simulink model "EKF_sim"  (R2020a)
settings: Solver=VariableStepAuto  StartTime=0.0  StopTime=257  RelTol=1e-3
values from neighbouring files (symbols this model uses):
  acc_variance = 4.8e-2    (= 0.048)    [init.m]
  bias_acc_variance = 4e-14    [init.m]
  bias_gyro_variance = 4e-14    [init.m]
  Delta2 = [260.168 -23.8158 1.64305]    [init.m]
  DT = EKF_DT    (= 0.01)    [init.m]
  EKF_DT = 0.01    [init.m]
  g = 9.81    [init.m]
  GPS_variance = 5    [init.m]
  gyro_variance = 4.8e-6    (= 4.8e-06)    [init.m]
  h0 = 38.8887000000000000    (= 38.8887)    [init.m]
  head_variance = 5e-2    (= 0.05)    [init.m]
  init_time = 4    [init.m]
  lambda_xa = 1e-4    (= 0.0001)    [init.m]
  lambda_xg = 1e-3    (= 0.001)    [init.m]
  lat0 = 36.7144590750000006    (= 36.714459075)    [init.m]
  lon0 = -4.4789588283333330    (= -4.47895882833)    [init.m]
  SHOE_buffer_N = 100    [init.m]
  SHOE_threshold = 2000    [init.m]
  t1_end = 100    [init.m]
  t1_start = 90    [init.m]
  t2_end = 193    [init.m]
  t2_start = 183    [init.m]
  t3_end = 213    [init.m]
  t3_start = 203    [init.m]
  t4_end = 244    [init.m]
  t4_start = 237    [init.m]
  type_of_GPS = 1    [init.m]
  vel_variance = 1e-2    (= 0.01)    [init.m]
  zero_vel_period = 0.1    [init.m]
(part 1 of 5)
settings Model: PauseTimes=232.9  Creator=Marco  LastModifiedBy=Marco

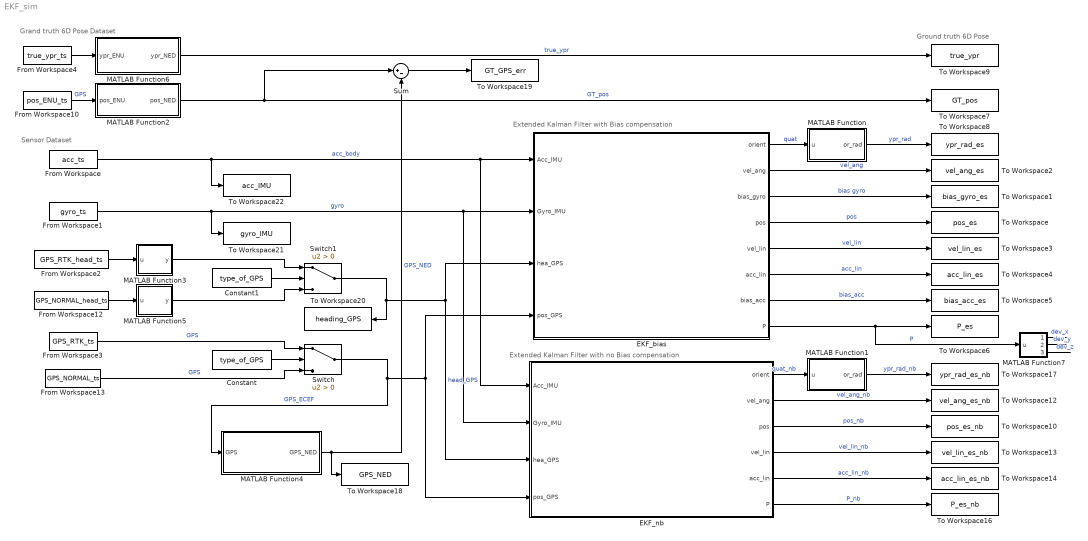
== system EKF_sim ==
  note: Grand truth 6D Pose Dataset
  note: Ground truth 6D Pose
  note: Sensor Dataset
  note: Extended Kalman Filter with Bias compensation
  note: Extended Kalman Filter with no Bias compensation
  Constant : Constant  Value=type_of_GPS
  Constant1 : Constant  Value=type_of_GPS
  EKF_bias : Subsystem
  EKF_nb : Subsystem
  From Workspace : FromWorkspace  VariableName=acc_ts  SampleTime=EKF_DT  OutputAfterFinalValue=Holding final value
  From Workspace1 : FromWorkspace  VariableName=gyro_ts  SampleTime=EKF_DT  OutputAfterFinalValue=Holding final value
  From Workspace10 : FromWorkspace  VariableName=pos_ENU_ts  SampleTime=0.01  OutputAfterFinalValue=Holding final value
  From Workspace12 : FromWorkspace  VariableName=GPS_NORMAL_head_ts  SampleTime=1  Interpolate=off  OutputAfterFinalValue=Holding final value
  From Workspace13 : FromWorkspace  VariableName=GPS_NORMAL_ts  SampleTime=1  Interpolate=off  OutputAfterFinalValue=Holding final value
  From Workspace2 : FromWorkspace  VariableName=GPS_RTK_head_ts  SampleTime=0.25  OutputAfterFinalValue=Holding final value
  From Workspace3 : FromWorkspace  VariableName=GPS_RTK_ts  SampleTime=0.25  OutputAfterFinalValue=Holding final value
  From Workspace4 : FromWorkspace  VariableName=true_ypr_ts  SampleTime=EKF_DT  OutputAfterFinalValue=Holding final value
  MATLAB Function : MATLAB Function  TreatAsAtomicUnit=on
  MATLAB Function1 : MATLAB Function  TreatAsAtomicUnit=on
  MATLAB Function2 : MATLAB Function  TreatAsAtomicUnit=on
  MATLAB Function3 : MATLAB Function  TreatAsAtomicUnit=on
  MATLAB Function4 : MATLAB Function  TreatAsAtomicUnit=on
  MATLAB Function5 : MATLAB Function  TreatAsAtomicUnit=on
  MATLAB Function6 : MATLAB Function  TreatAsAtomicUnit=on
  MATLAB Function7 : MATLAB Function  TreatAsAtomicUnit=on
  Sum : Sum  Inputs=|+-
  Switch : Switch  Criteria=u2 > Threshold
  Switch1 : Switch  Criteria=u2 > Threshold
  To Workspace : ToWorkspace  VariableName=pos_es  SaveFormat=Timeseries  SampleTime=-1
  To Workspace1 : ToWorkspace  VariableName=bias_gyro_es  SaveFormat=Timeseries  SampleTime=-1
  To Workspace10 : ToWorkspace  VariableName=pos_es_nb  SaveFormat=Timeseries  SampleTime=-1
  To Workspace12 : ToWorkspace  VariableName=vel_ang_es_nb  SaveFormat=Timeseries  SampleTime=-1
  To Workspace13 : ToWorkspace  VariableName=vel_lin_es_nb  SaveFormat=Timeseries  SampleTime=-1
  To Workspace14 : ToWorkspace  VariableName=acc_lin_es_nb  SaveFormat=Timeseries  SampleTime=-1
  To Workspace16 : ToWorkspace  VariableName=P_es_nb  SaveFormat=Timeseries  SampleTime=-1
  To Workspace17 : ToWorkspace  VariableName=ypr_rad_es_nb  SaveFormat=Timeseries  SampleTime=-1
  To Workspace18 : ToWorkspace  VariableName=GPS_NED  SaveFormat=Timeseries  SampleTime=-1
  To Workspace19 : ToWorkspace  VariableName=GT_GPS_err  SaveFormat=Timeseries  SampleTime=-1
  To Workspace2 : ToWorkspace  VariableName=vel_ang_es  SaveFormat=Timeseries  SampleTime=-1
  To Workspace20 : ToWorkspace  VariableName=heading_GPS  SaveFormat=Timeseries  SampleTime=-1
  To Workspace21 : ToWorkspace  VariableName=gyro_IMU  SaveFormat=Timeseries  SampleTime=-1
  To Workspace22 : ToWorkspace  VariableName=acc_IMU  SaveFormat=Timeseries  SampleTime=-1
  To Workspace3 : ToWorkspace  VariableName=vel_lin_es  SaveFormat=Timeseries  SampleTime=-1
  To Workspace4 : ToWorkspace  VariableName=acc_lin_es  SaveFormat=Timeseries  SampleTime=-1
  To Workspace5 : ToWorkspace  VariableName=bias_acc_es  SaveFormat=Timeseries  SampleTime=-1
  To Workspace6 : ToWorkspace  VariableName=P_es  SaveFormat=Timeseries  SampleTime=-1
  To Workspace7 : ToWorkspace  VariableName=GT_pos  SaveFormat=Timeseries  SampleTime=-1
  To Workspace8 : ToWorkspace  VariableName=ypr_rad_es  SaveFormat=Timeseries  SampleTime=-1
  To Workspace9 : ToWorkspace  VariableName=true_ypr  SaveFormat=Timeseries  SampleTime=-1
  wires:
  EKF_bias/4(pos) -> To Workspace/1  "pos"
  EKF_bias/1(orient) -> MATLAB Function/1(u)  "quat"
  EKF_bias/2(vel_ang) -> To Workspace2/1  "vel_ang"
  EKF_bias/3(bias_gyro) -> To Workspace1/1  "bias gyro"
  EKF_bias/6(acc_lin) -> To Workspace4/1  "acc_lin"
  EKF_bias/7(bias_acc) -> To Workspace5/1  "bias_acc"
  EKF_bias/8(P) -> MATLAB Function7/1(u), To Workspace6/1  "P"
  MATLAB Function/1(or_rad) -> To Workspace8/1  "ypr_rad"
  From Workspace/1 -> To Workspace22/1, EKF_nb/1(Acc_IMU), EKF_bias/1(Acc_IMU)  "acc_body"
  From Workspace1/1 -> To Workspace21/1, EKF_nb/2(Gyro_IMU), EKF_bias/2(Gyro_IMU)  "gyro"
  From Workspace4/1 -> MATLAB Function6/1(ypr_ENU)
  MATLAB Function6/1(ypr_NED) -> To Workspace9/1  "true_ypr"
  From Workspace10/1 -> MATLAB Function2/1(pos_ENU)  "GPS"
  MATLAB Function2/1(pos_NED) -> To Workspace7/1, Sum/1  "GT_pos"
  EKF_bias/5(vel_lin) -> To Workspace3/1  "vel_lin"
  Constant/1 -> Switch/2
  From Workspace2/1 -> MATLAB Function3/1(u)
  From Workspace3/1 -> Switch/1  "GPS"
  MATLAB Function3/1(y) -> Switch1/1
  Constant1/1 -> Switch1/2
  Switch1/1 -> To Workspace20/1, EKF_bias/3(hea_GPS), EKF_nb/3(hea_GPS)  "head_GPS"
  Switch/1 -> MATLAB Function4/1(GPS), EKF_nb/4(pos_GPS), EKF_bias/4(pos_GPS)  "GPS_ECEF"
  From Workspace12/1 -> MATLAB Function5/1(u)
  MATLAB Function5/1(y) -> Switch1/3
  From Workspace13/1 -> Switch/3  "GPS"
  EKF_nb/4(vel_lin) -> To Workspace13/1  "vel_lin_nb"
  MATLAB Function1/1(or_rad) -> To Workspace17/1  "ypr_rad_nb"
  EKF_nb/6(P) -> To Workspace16/1  "P_nb"
  EKF_nb/5(acc_lin) -> To Workspace14/1  "acc_lin_nb"
  EKF_nb/2(vel_ang) -> To Workspace12/1  "vel_ang_nb"
  EKF_nb/1(orient) -> MATLAB Function1/1(u)  "quat_nb"
  EKF_nb/3(pos) -> To Workspace10/1  "pos_nb"
  MATLAB Function4/1(GPS_NED) -> To Workspace18/1, Sum/2  "GPS_NED"
  Sum/1 -> To Workspace19/1
  MATLAB Function7/1(dev_x) -> ?  "dev_x"
  MATLAB Function7/2(dev_y) -> ?  "dev_y"
  MATLAB Function7/3(dev_z) -> ?  "dev_z"

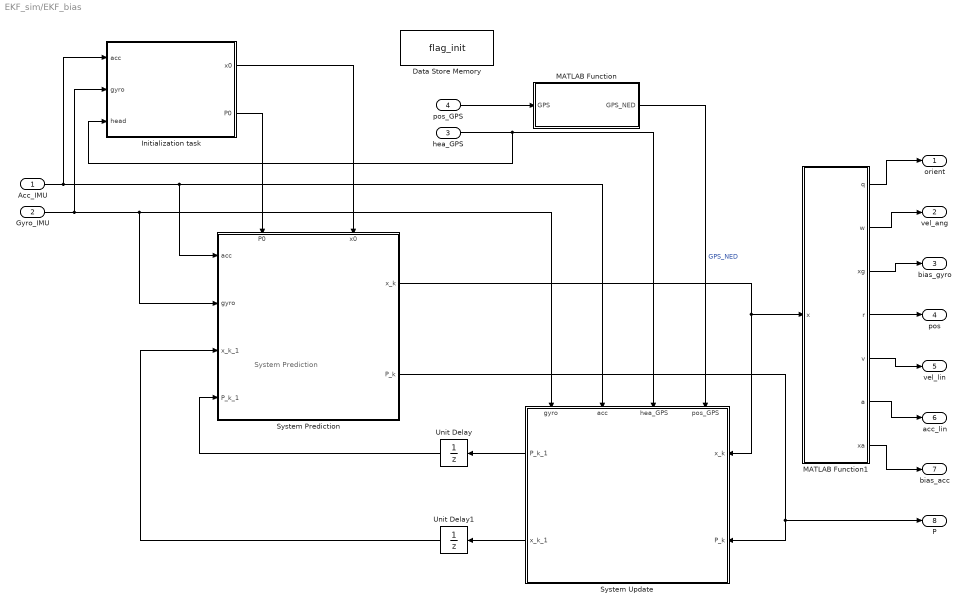
== system EKF_sim/EKF_bias ==
  note: System Prediction
  Acc_IMU : Inport
  Gyro_IMU : Inport  Port=2
  hea_GPS : Inport  Port=3
  pos_GPS : Inport  Port=4
  Data Store Memory : DataStoreMemory  DataStoreName=flag_init  InitialValue=-1  ShowAdditionalParam=off
  Initialization task : Subsystem
  MATLAB Function : MATLAB Function  TreatAsAtomicUnit=on
  MATLAB Function1 : MATLAB Function  TreatAsAtomicUnit=on
  System Prediction : Subsystem
      settings: PortSchema="{\"entries\":[{\"content\":{\"sides\":[{\"content\":{\"connectorIds\":[\"In1\",\"In2\",\"In3\",\"In4\"]},\"type\":\"ConnectorPlacement.EquallySpacedRectSide\",\"uuid\":\"a31c1247-8445-41f9-872e-e95041ac67e2\"},{\"content\":{\"connectorIds\":[\"Out1\",\"Out2\"],\"side\":\"RIGHT\"},\"type\":\"ConnectorPlacement.EquallySpacedRectSide\",\"uuid\":\"88e5873f-61bb-437e-a1ee-da954a8709d0\"},{\"content\":{\"connectorIds\":[\"In5\",\"In6\"],\"side\":\"TOP\"},\"type\":\"ConnectorPlacement.EquallySpacedRectSide\",\"uuid\":\"ffd70c81-5e0f-418c-96ba-bca8f59ed82d\"}]},\"type\":\"ConnectorPlacement.EquallySpacedConnector\",\"uuid\":\"15174104-45ca-4697-baa5-649374845b9a\"}],\"packageUris\":[\"http://schema.mathworks.com/mf0/Connector/19700101\"],\"version\":\"1.0\"}"
  System Update : Subsystem
      settings: PortSchema="{\"entries\":[{\"content\":{\"sides\":[{\"content\":{\"connectorIds\":[\"In1\",\"In2\"]},\"type\":\"ConnectorPlacement.EquallySpacedRectSide\",\"uuid\":\"5c80ded8-dd2e-4acc-ae6d-b7377cd46508\"},{\"content\":{\"connectorIds\":[\"Out1\",\"Out2\"],\"side\":\"RIGHT\"},\"type\":\"ConnectorPlacement.EquallySpacedRectSide\",\"uuid\":\"972e6236-a0c8-4bf9-b48b-7617d612a7cb\"},{\"content\":{\"connectorIds\":[\"In3\",\"In4\",\"In5\",\"In6\"],\"side\":\"TOP\"},\"type\":\"ConnectorPlacement.EquallySpacedRectSide\",\"uuid\":\"226aceb0-2664-4cce-b0bd-7f8238cad43e\"}]},\"type\":\"ConnectorPlacement.EquallySpacedConnector\",\"uuid\":\"4d3b7443-5747-48ca-9145-cac0c7b86d89\"}],\"packageUris\":[\"http://schema.mathworks.com/mf0/Connector/19700101\"],\"version\":\"1.0\"}"
  Unit Delay : UnitDelay  SampleTime=-1  HasFrameUpgradeWarning=on
  Unit Delay1 : UnitDelay  SampleTime=-1  HasFrameUpgradeWarning=on
  orient : Outport
  vel_ang : Outport  Port=2
  bias_gyro : Outport  Port=3
  pos : Outport  Port=4
  vel_lin : Outport  Port=5
  acc_lin : Outport  Port=6
  bias_acc : Outport  Port=7
  P : Outport  Port=8
  wires:
  MATLAB Function1/7(xa) -> bias_acc/1
  MATLAB Function1/6(a) -> acc_lin/1
  MATLAB Function1/5(v) -> vel_lin/1
  MATLAB Function1/4(r) -> pos/1
  MATLAB Function1/3(xg) -> bias_gyro/1
  MATLAB Function1/2(w) -> vel_ang/1
  MATLAB Function1/1(q) -> orient/1
  System Prediction/2(P_k) -> P/1, System Update/2(P_k)
  System Prediction/1(x_k) -> MATLAB Function1/1(x), System Update/1(x_k)
  System Update/1(P_k_1) -> Unit Delay/1
  System Update/2(x_k_1) -> Unit Delay1/1
  hea_GPS/1 -> Initialization task/3(head), System Update/4(hea_GPS)
  MATLAB Function/1(GPS_NED) -> System Update/3(pos_GPS)  "GPS_NED"
  pos_GPS/1 -> MATLAB Function/1(GPS)
  Initialization task/1(x0) -> System Prediction/6(x0)
  Initialization task/2(P0) -> System Prediction/5(P0)
  Gyro_IMU/1 -> Initialization task/2(gyro), System Prediction/2(gyro), System Update/6(gyro)
  Acc_IMU/1 -> Initialization task/1(acc), System Update/5(acc), System Prediction/1(acc)
  Unit Delay/1 -> System Prediction/4(P_k_1)
  Unit Delay1/1 -> System Prediction/3(x_k_1)

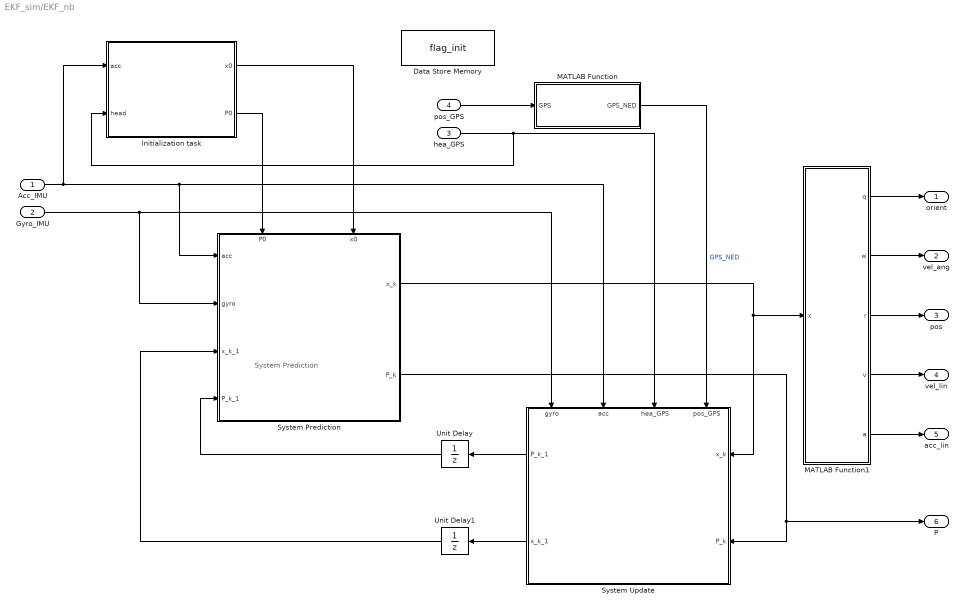
== system EKF_sim/EKF_nb ==
  note: System Prediction
  Acc_IMU : Inport
  Gyro_IMU : Inport  Port=2
  hea_GPS : Inport  Port=3
  pos_GPS : Inport  Port=4
  Data Store Memory : DataStoreMemory  DataStoreName=flag_init  InitialValue=-1  ShowAdditionalParam=off
  Initialization task : Subsystem
  MATLAB Function : MATLAB Function  TreatAsAtomicUnit=on
  MATLAB Function1 : MATLAB Function  TreatAsAtomicUnit=on
  System Prediction : Subsystem
      settings: PortSchema="{\"entries\":[{\"content\":{\"sides\":[{\"content\":{\"connectorIds\":[\"In1\",\"In2\",\"In3\",\"In4\"]},\"type\":\"ConnectorPlacement.EquallySpacedRectSide\",\"uuid\":\"a31c1247-8445-41f9-872e-e95041ac67e2\"},{\"content\":{\"connectorIds\":[\"Out1\",\"Out2\"],\"side\":\"RIGHT\"},\"type\":\"ConnectorPlacement.EquallySpacedRectSide\",\"uuid\":\"88e5873f-61bb-437e-a1ee-da954a8709d0\"},{\"content\":{\"connectorIds\":[\"In5\",\"In6\"],\"side\":\"TOP\"},\"type\":\"ConnectorPlacement.EquallySpacedRectSide\",\"uuid\":\"ffd70c81-5e0f-418c-96ba-bca8f59ed82d\"}]},\"type\":\"ConnectorPlacement.EquallySpacedConnector\",\"uuid\":\"15174104-45ca-4697-baa5-649374845b9a\"}],\"packageUris\":[\"http://schema.mathworks.com/mf0/Connector/19700101\"],\"version\":\"1.0\"}"
  System Update : Subsystem
      settings: PortSchema="{\"entries\":[{\"content\":{\"sides\":[{\"content\":{\"connectorIds\":[\"In1\",\"In2\"]},\"type\":\"ConnectorPlacement.EquallySpacedRectSide\",\"uuid\":\"5c80ded8-dd2e-4acc-ae6d-b7377cd46508\"},{\"content\":{\"connectorIds\":[\"Out1\",\"Out2\"],\"side\":\"RIGHT\"},\"type\":\"ConnectorPlacement.EquallySpacedRectSide\",\"uuid\":\"972e6236-a0c8-4bf9-b48b-7617d612a7cb\"},{\"content\":{\"connectorIds\":[\"In3\",\"In4\",\"In5\",\"In6\"],\"side\":\"TOP\"},\"type\":\"ConnectorPlacement.EquallySpacedRectSide\",\"uuid\":\"226aceb0-2664-4cce-b0bd-7f8238cad43e\"}]},\"type\":\"ConnectorPlacement.EquallySpacedConnector\",\"uuid\":\"4d3b7443-5747-48ca-9145-cac0c7b86d89\"}],\"packageUris\":[\"http://schema.mathworks.com/mf0/Connector/19700101\"],\"version\":\"1.0\"}"
  Unit Delay : UnitDelay  SampleTime=-1  HasFrameUpgradeWarning=on
  Unit Delay1 : UnitDelay  SampleTime=-1  HasFrameUpgradeWarning=on
  orient : Outport
  vel_ang : Outport  Port=2
  pos : Outport  Port=3
  vel_lin : Outport  Port=4
  acc_lin : Outport  Port=5
  P : Outport  Port=6
  wires:
  Unit Delay1/1 -> System Prediction/3(x_k_1)
  Unit Delay/1 -> System Prediction/4(P_k_1)
  Acc_IMU/1 -> System Prediction/1(acc), System Update/5(acc), Initialization task/1(acc)
  Gyro_IMU/1 -> System Update/6(gyro), System Prediction/2(gyro)
  Initialization task/2(P0) -> System Prediction/5(P0)
  Initialization task/1(x0) -> System Prediction/6(x0)
  pos_GPS/1 -> MATLAB Function/1(GPS)
  MATLAB Function/1(GPS_NED) -> System Update/3(pos_GPS)  "GPS_NED"
  hea_GPS/1 -> System Update/4(hea_GPS), Initialization task/2(head)
  System Update/2(x_k_1) -> Unit Delay1/1
  System Update/1(P_k_1) -> Unit Delay/1
  System Prediction/1(x_k) -> System Update/1(x_k), MATLAB Function1/1(x)
  System Prediction/2(P_k) -> System Update/2(P_k), P/1
  MATLAB Function1/1(q) -> orient/1
  MATLAB Function1/2(w) -> vel_ang/1
  MATLAB Function1/3(r) -> pos/1
  MATLAB Function1/4(v) -> vel_lin/1
  MATLAB Function1/5(a) -> acc_lin/1

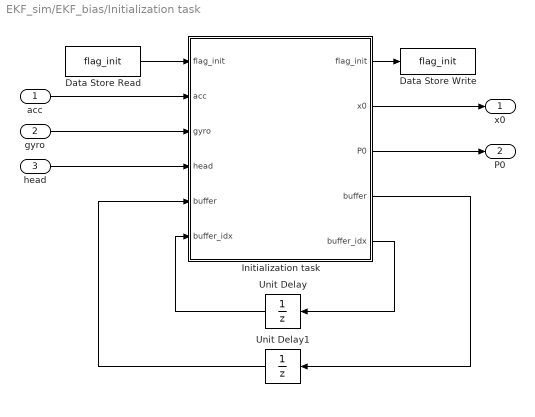
== system EKF_sim/EKF_bias/Initialization task ==
  acc : Inport
  gyro : Inport  Port=2
  head : Inport  Port=3
  Data Store Read : DataStoreRead  DataStoreName=flag_init  DataStoreElements=flag_init
  Data Store Write : DataStoreWrite  DataStoreName=flag_init  DataStoreElements=flag_init
  Initialization task : MATLAB Function  TreatAsAtomicUnit=on  SystemSampleTime=EKF_DT
  Unit Delay : UnitDelay  InitialCondition=1  SampleTime=-1  HasFrameUpgradeWarning=on
  Unit Delay1 : UnitDelay  InitialCondition=zeros(100*init_time,7)  SampleTime=-1  HasFrameUpgradeWarning=on
  x0 : Outport
  P0 : Outport  Port=2
  wires:
  Initialization task/1(flag_init) -> Data Store Write/1
  Data Store Read/1 -> Initialization task/1("flag_init ")
  Initialization task/2(x0) -> x0/1
  Initialization task/3(P0) -> P0/1
  acc/1 -> Initialization task/2(acc)
  gyro/1 -> Initialization task/3(gyro)
  Initialization task/4(buffer) -> Unit Delay1/1
  Initialization task/5(buffer_idx) -> Unit Delay/1
  Unit Delay/1 -> Initialization task/6("buffer_idx ")
  head/1 -> Initialization task/4(head)
  Unit Delay1/1 -> Initialization task/5("buffer ")

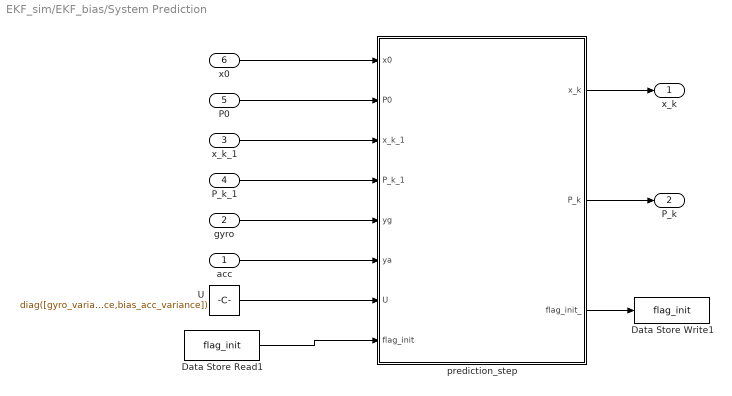
== system EKF_sim/EKF_bias/System Prediction ==
  acc : Inport
  gyro : Inport  Port=2
  x_k_1 : Inport  Port=3
  P_k_1 : Inport  Port=4
  P0 : Inport  Port=5
  x0 : Inport  Port=6
  Data Store Read1 : DataStoreRead  DataStoreName=flag_init  DataStoreElements=flag_init
  Data Store Write1 : DataStoreWrite  DataStoreName=flag_init  DataStoreElements=flag_init
  U : Constant  Value=diag([gyro_variance,gyro_variance,gyro_variance,bias_gyro_variance,bias_gyro_variance,bias_gyro_variance,acc_variance,acc_variance,acc_variance,bias_acc_variance,bias_acc_variance,bias_acc_variance])  VectorParams1D=off
  prediction_step : MATLAB Function  TreatAsAtomicUnit=on  SystemSampleTime=EKF_DT
  x_k : Outport
  P_k : Outport  Port=2
  wires:
  prediction_step/2(P_k) -> P_k/1
  prediction_step/1(x_k) -> x_k/1
  x_k_1/1 -> prediction_step/3(x_k_1)
  P_k_1/1 -> prediction_step/4(P_k_1)
  gyro/1 -> prediction_step/5(yg)
  acc/1 -> prediction_step/6(ya)
  U/1 -> prediction_step/7(U)
  Data Store Read1/1 -> prediction_step/8(flag_init)
  prediction_step/3(flag_init_) -> Data Store Write1/1
  x0/1 -> prediction_step/1(x0)
  P0/1 -> prediction_step/2(P0)

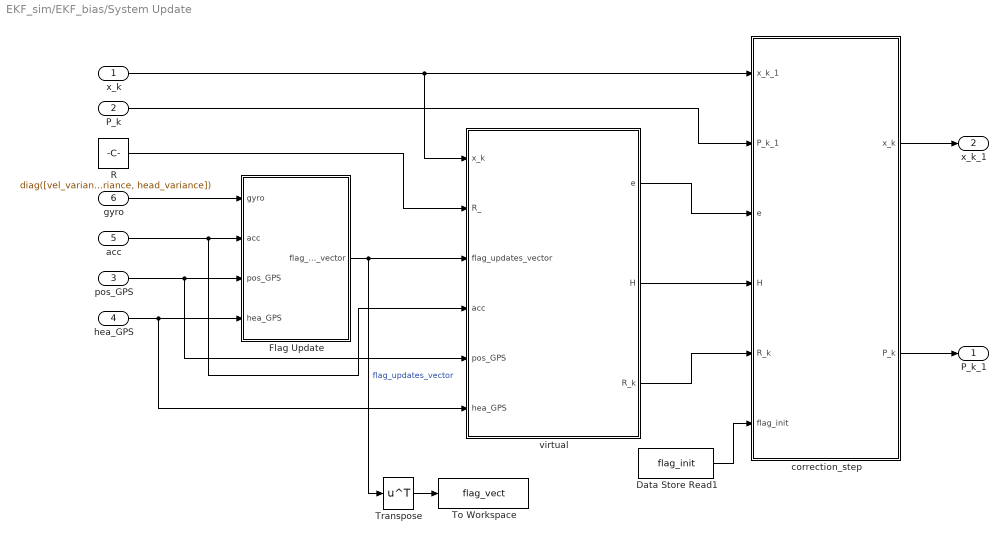
== system EKF_sim/EKF_bias/System Update ==
  x_k : Inport
  P_k : Inport  Port=2
  pos_GPS : Inport  Port=3
  hea_GPS : Inport  Port=4
  acc : Inport  Port=5
  gyro : Inport  Port=6
  Data Store Read1 : DataStoreRead  DataStoreName=flag_init  DataStoreElements=flag_init
  Flag Update : Subsystem
  R : Constant  Value=diag([vel_variance,vel_variance, acc_variance, acc_variance, acc_variance, GPS_variance, GPS_variance, GPS_variance, head_variance])  VectorParams1D=off
  To Workspace : ToWorkspace  VariableName=flag_vect  SaveFormat=Timeseries  SampleTime=-1
  Transpose : Math  Operator=transpose  SaturateOnIntegerOverflow=on
  correction_step : MATLAB Function  TreatAsAtomicUnit=on  SystemSampleTime=EKF_DT
  virtual : MATLAB Function  TreatAsAtomicUnit=on  SystemSampleTime=EKF_DT
  P_k_1 : Outport
  x_k_1 : Outport  Port=2
  wires:
  x_k/1 -> correction_step/1(x_k_1), virtual/1(x_k)
  correction_step/1(x_k) -> x_k_1/1
  correction_step/2(P_k) -> P_k_1/1
  P_k/1 -> correction_step/2(P_k_1)
  virtual/1(e) -> correction_step/3(e)
  virtual/2(H) -> correction_step/4(H)
  virtual/3(R_k) -> correction_step/5(R_k)
  R/1 -> virtual/2(R_)
  hea_GPS/1 -> virtual/6(hea_GPS), Flag Update/4(hea_GPS)
  pos_GPS/1 -> virtual/5(pos_GPS), Flag Update/3(pos_GPS)
  acc/1 -> Flag Update/2(acc), virtual/4(acc)
  gyro/1 -> Flag Update/1(gyro)
  Flag Update/1(flag_updates_vector) -> virtual/3(flag_updates_vector), Transpose/1  "flag_updates_vector"
  Data Store Read1/1 -> correction_step/6(flag_init)
  Transpose/1 -> To Workspace/1

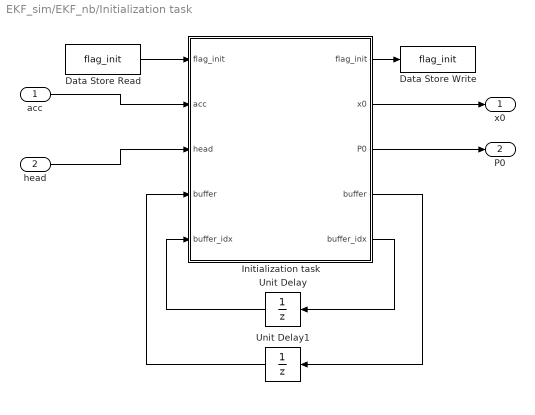
== system EKF_sim/EKF_nb/Initialization task ==
  acc : Inport
  head : Inport  Port=2
  Data Store Read : DataStoreRead  DataStoreName=flag_init  DataStoreElements=flag_init
  Data Store Write : DataStoreWrite  DataStoreName=flag_init  DataStoreElements=flag_init
  Initialization task : MATLAB Function  TreatAsAtomicUnit=on  SystemSampleTime=EKF_DT
  Unit Delay : UnitDelay  InitialCondition=1  SampleTime=-1  HasFrameUpgradeWarning=on
  Unit Delay1 : UnitDelay  InitialCondition=zeros(100*init_time,4)  SampleTime=-1  HasFrameUpgradeWarning=on
  x0 : Outport
  P0 : Outport  Port=2
  wires:
  Unit Delay1/1 -> Initialization task/4("buffer ")
  head/1 -> Initialization task/3(head)
  Unit Delay/1 -> Initialization task/5("buffer_idx ")
  Initialization task/5(buffer_idx) -> Unit Delay/1
  Initialization task/4(buffer) -> Unit Delay1/1
  acc/1 -> Initialization task/2(acc)
  Initialization task/3(P0) -> P0/1
  Initialization task/2(x0) -> x0/1
  Data Store Read/1 -> Initialization task/1("flag_init ")
  Initialization task/1(flag_init) -> Data Store Write/1

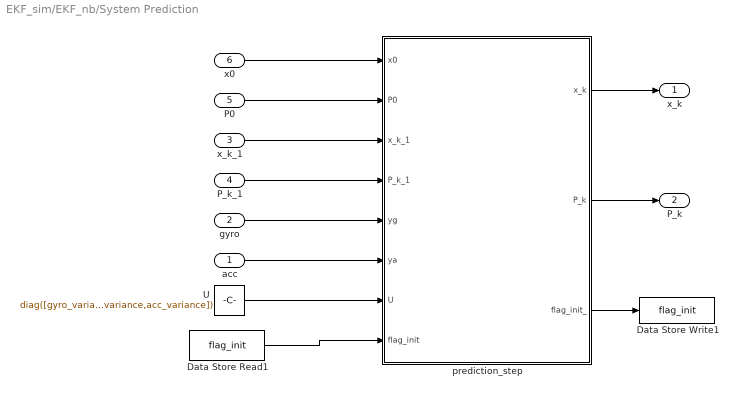
== system EKF_sim/EKF_nb/System Prediction ==
  acc : Inport
  gyro : Inport  Port=2
  x_k_1 : Inport  Port=3
  P_k_1 : Inport  Port=4
  P0 : Inport  Port=5
  x0 : Inport  Port=6
  Data Store Read1 : DataStoreRead  DataStoreName=flag_init  DataStoreElements=flag_init
  Data Store Write1 : DataStoreWrite  DataStoreName=flag_init  DataStoreElements=flag_init
  U : Constant  Value=diag([gyro_variance,gyro_variance,gyro_variance,acc_variance,acc_variance,acc_variance])  VectorParams1D=off
  prediction_step : MATLAB Function  TreatAsAtomicUnit=on  SystemSampleTime=EKF_DT
  x_k : Outport
  P_k : Outport  Port=2
  wires:
  P0/1 -> prediction_step/2(P0)
  x0/1 -> prediction_step/1(x0)
  prediction_step/3(flag_init_) -> Data Store Write1/1
  Data Store Read1/1 -> prediction_step/8(flag_init)
  U/1 -> prediction_step/7(U)
  acc/1 -> prediction_step/6(ya)
  gyro/1 -> prediction_step/5(yg)
  P_k_1/1 -> prediction_step/4(P_k_1)
  x_k_1/1 -> prediction_step/3(x_k_1)
  prediction_step/1(x_k) -> x_k/1
  prediction_step/2(P_k) -> P_k/1

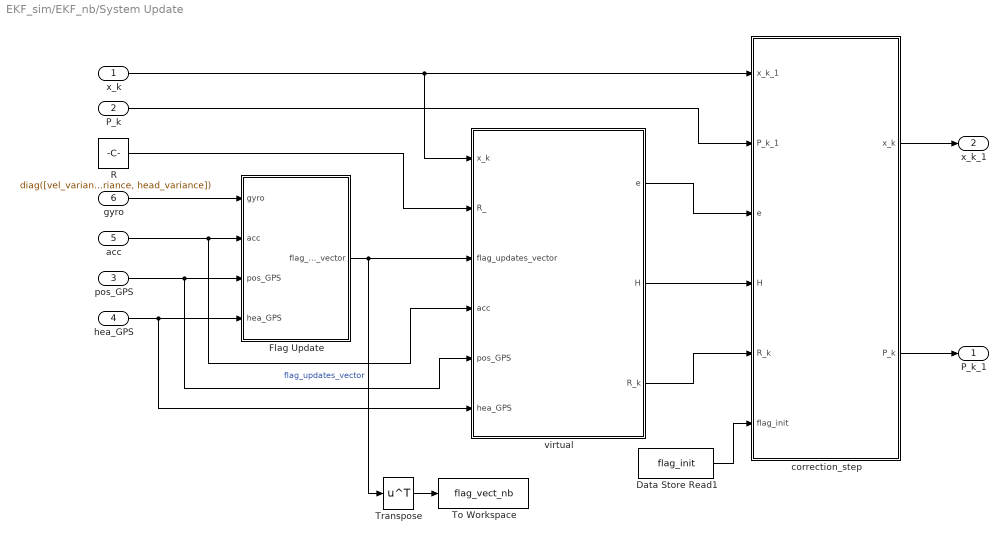
== system EKF_sim/EKF_nb/System Update ==
  x_k : Inport
  P_k : Inport  Port=2
  pos_GPS : Inport  Port=3
  hea_GPS : Inport  Port=4
  acc : Inport  Port=5
  gyro : Inport  Port=6
  Data Store Read1 : DataStoreRead  DataStoreName=flag_init  DataStoreElements=flag_init
  Flag Update : Subsystem
  R : Constant  Value=diag([vel_variance,vel_variance, acc_variance, acc_variance, acc_variance, GPS_variance, GPS_variance, GPS_variance, head_variance])  VectorParams1D=off
  To Workspace : ToWorkspace  VariableName=flag_vect_nb  SaveFormat=Timeseries  SampleTime=-1
  Transpose : Math  Operator=transpose  SaturateOnIntegerOverflow=on
  correction_step : MATLAB Function  TreatAsAtomicUnit=on  SystemSampleTime=EKF_DT
  virtual : MATLAB Function  TreatAsAtomicUnit=on  SystemSampleTime=EKF_DT
  P_k_1 : Outport
  x_k_1 : Outport  Port=2
  wires:
  Transpose/1 -> To Workspace/1
  Data Store Read1/1 -> correction_step/6(flag_init)
  Flag Update/1(flag_updates_vector) -> Transpose/1, virtual/3(flag_updates_vector)  "flag_updates_vector"
  gyro/1 -> Flag Update/1(gyro)
  acc/1 -> virtual/4(acc), Flag Update/2(acc)
  pos_GPS/1 -> Flag Update/3(pos_GPS), virtual/5(pos_GPS)
  hea_GPS/1 -> Flag Update/4(hea_GPS), virtual/6(hea_GPS)
  R/1 -> virtual/2(R_)
  virtual/3(R_k) -> correction_step/5(R_k)
  virtual/2(H) -> correction_step/4(H)
  virtual/1(e) -> correction_step/3(e)
  P_k/1 -> correction_step/2(P_k_1)
  correction_step/2(P_k) -> P_k_1/1
  correction_step/1(x_k) -> x_k_1/1
  x_k/1 -> virtual/1(x_k), correction_step/1(x_k_1)

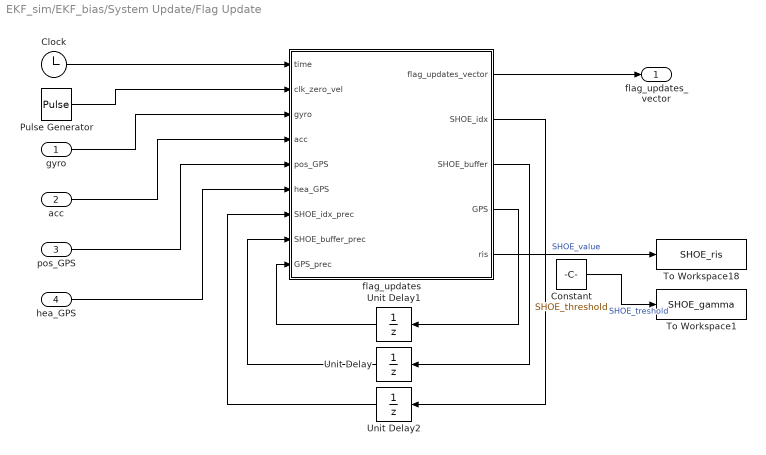
== system EKF_sim/EKF_bias/System Update/Flag Update ==
  gyro : Inport
  acc : Inport  Port=2
  pos_GPS : Inport  Port=3
  hea_GPS : Inport  Port=4
  Clock : Clock
  Constant : Constant  Value=SHOE_threshold
  Pulse Generator : DiscretePulseGenerator  PulseType=Time based  Period=zero_vel_period  PhaseDelay=zero_vel_period
  To Workspace1 : ToWorkspace  VariableName=SHOE_gamma  SaveFormat=Timeseries  SampleTime=-1
  To Workspace18 : ToWorkspace  VariableName=SHOE_ris  SaveFormat=Timeseries  SampleTime=-1
  Unit Delay : UnitDelay  InitialCondition=zeros(SHOE_buffer_N,6)  SampleTime=-1  HasFrameUpgradeWarning=on
  Unit Delay1 : UnitDelay  InitialCondition=[0 0 0 0]  SampleTime=-1  HasFrameUpgradeWarning=on
  Unit Delay2 : UnitDelay  InitialCondition=1  SampleTime=-1  HasFrameUpgradeWarning=on
  flag_updates : MATLAB Function  TreatAsAtomicUnit=on  SystemSampleTime=EKF_DT
  flag_updates_vector : Outport
  wires:
  Unit Delay1/1 -> flag_updates/9(GPS_prec)
  acc/1 -> flag_updates/4(acc)
  Pulse Generator/1 -> flag_updates/2(clk_zero_vel)
  flag_updates/4(GPS) -> Unit Delay1/1
  Unit Delay/1 -> flag_updates/8(SHOE_buffer_prec)
  hea_GPS/1 -> flag_updates/6(hea_GPS)
  flag_updates/3(SHOE_buffer) -> Unit Delay/1
  flag_updates/2(SHOE_idx) -> Unit Delay2/1
  Unit Delay2/1 -> flag_updates/7(SHOE_idx_prec)
  pos_GPS/1 -> flag_updates/5(pos_GPS)
  gyro/1 -> flag_updates/3(gyro)
  flag_updates/1(flag_updates_vector) -> flag_updates_vector/1
  flag_updates/5(ris) -> To Workspace18/1  "SHOE_value"
  Constant/1 -> To Workspace1/1  "SHOE_treshold"
  Clock/1 -> flag_updates/1(time)

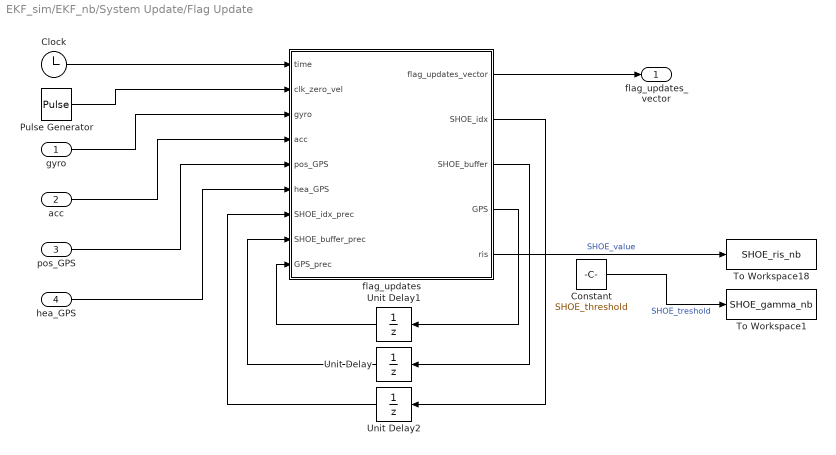
== system EKF_sim/EKF_nb/System Update/Flag Update ==
  gyro : Inport
  acc : Inport  Port=2
  pos_GPS : Inport  Port=3
  hea_GPS : Inport  Port=4
  Clock : Clock
  Constant : Constant  Value=SHOE_threshold
  Pulse Generator : DiscretePulseGenerator  PulseType=Time based  Period=zero_vel_period  PhaseDelay=zero_vel_period
  To Workspace1 : ToWorkspace  VariableName=SHOE_gamma_nb  SaveFormat=Timeseries  SampleTime=-1
  To Workspace18 : ToWorkspace  VariableName=SHOE_ris_nb  SaveFormat=Timeseries  SampleTime=-1
  Unit Delay : UnitDelay  InitialCondition=zeros(SHOE_buffer_N,6)  SampleTime=-1  HasFrameUpgradeWarning=on
  Unit Delay1 : UnitDelay  InitialCondition=[0 0 0 0]  SampleTime=-1  HasFrameUpgradeWarning=on
  Unit Delay2 : UnitDelay  InitialCondition=1  SampleTime=-1  HasFrameUpgradeWarning=on
  flag_updates : MATLAB Function  TreatAsAtomicUnit=on  SystemSampleTime=EKF_DT
  flag_updates_vector : Outport
  wires:
  Clock/1 -> flag_updates/1(time)
  Constant/1 -> To Workspace1/1  "SHOE_treshold"
  flag_updates/5(ris) -> To Workspace18/1  "SHOE_value"
  flag_updates/1(flag_updates_vector) -> flag_updates_vector/1
  gyro/1 -> flag_updates/3(gyro)
  pos_GPS/1 -> flag_updates/5(pos_GPS)
  Unit Delay2/1 -> flag_updates/7(SHOE_idx_prec)
  flag_updates/2(SHOE_idx) -> Unit Delay2/1
  flag_updates/3(SHOE_buffer) -> Unit Delay/1
  hea_GPS/1 -> flag_updates/6(hea_GPS)
  Unit Delay/1 -> flag_updates/8(SHOE_buffer_prec)
  flag_updates/4(GPS) -> Unit Delay1/1
  Pulse Generator/1 -> flag_updates/2(clk_zero_vel)
  acc/1 -> flag_updates/4(acc)
  Unit Delay1/1 -> flag_updates/9(GPS_prec)

== matlab function EKF_sim/EKF_bias/System Update/correction_step ==
  data: x_k_1 input; x_k output; P_k_1 input; e input size=9 1; H input size=9 22; R_k input size=9 9; P_k output; flag_init input
% --------------------         correction           -------------------- %
%{
% This function computes the correction step of the Kalman Filter. When new
% updates are avaiable, the Kalman Gain is updated and the vector state and
% matrix P too.

% Input:
%     x_k_1     : [22x1] state vector before correction step
%     P_k_1     : [22x22] matrix P before correction step
%     e         : [] Error between current measure and predicted measure
%     H         : [] Jacobian of prediction model measurement with respect 
%                 to state x
%     R_k       : [] Measurement Noise Covariance Matrix at time k
%     flag_init : flag for initialization task

% Output:
%     x_k       : [22x1] state vector after correction step
%     P_k       : [22x22] matrix P after correction step

% The formulas are?
%     S_k = H*P_k_1*H' + R_k;
%     K_k = P_k_1*H'*(inv(S_k));
%     P_k = (eye(22)-(K_k*H))*P_k_1;         
%     x_k = x_k_1 + K_k * e;
%}
%%
function [x_k, P_k] = correction(x_k_1, P_k_1, ...
                                 e, H, R_k, flag_init)
     x_k = zeros(22,1);
     P_k = zeros(22,22);
     
     if flag_init ~= -1
                
          S_k = H*P_k_1*H' + R_k;
          K_k = P_k_1*H'*(inv(S_k));

          P_k = (eye(22)-(K_k*H))*P_k_1;         
          x_k = x_k_1 + K_k * e;
     end
end

%% %%%%%%%%%%%%%%%%%%%%%%%%%%%%%%%%%%%%%%%%%%%%%%%%%%%%%%%%%%%%%%%%%%%%%%%
     %%%%%%%%% Direct EKF for 6D Pose,  Marco Borraccino %%%%%%%%%%
     %%%%%%%%%   SGN Project, University of Pisa, 2021   %%%%%%%%%%
%%%%%%%%%%%%%%%%%%%%%%%%%%%%%%%%%%%%%%%%%%%%%%%%%%%%%%%%%%%%%%%%%%%%%%%%%%

== matlab function EKF_sim/EKF_bias/MATLAB Function1 ==
  data: x input; q output; w output; xg output; r output; v output; a output; xa output
% --------------------         extract_var         -------------------- %
%{
% This function extracts single variables from the state vector.

% Input:
%     x  :  [q w xg r v a xa]' state vector [22x1]:

% Output:
%     q  : [q1 q2 q3 q4]     unit quaternion representing the attitude (1 2 3 4)
%     w  : [wx wy wz]        angular velocity (5 6 7)
%     xg : [xg_x xg_y xg_z]  gyro bias (8 9 10)
%     r  : [rx ry rz]        position (NED)(11 12 13)
%     v  : [vx vy vz]        linear velocity (NED) (14 15 16)
%     a  : [ax ay az]        linear acceleration (NED) (17 18 19)
%     xa : [xa_x xa_y xa_z]  accelerometer bias (20 21 22)
%}
%%
function [q, w,  xg, r, v, a, xa] = extract_var(x)
    q  = x(1:4);
    w  = x(5:7);
    xg = x(8:10);
    r  = x(11:13);
    v  = x(14:16);
    a  = x(17:19);
    xa = x(20:22);
end

%% %%%%%%%%%%%%%%%%%%%%%%%%%%%%%%%%%%%%%%%%%%%%%%%%%%%%%%%%%%%%%%%%%%%%%%%
     %%%%%%%%% Direct EKF for 6D Pose,  Marco Borraccino %%%%%%%%%%
     %%%%%%%%%   SGN Project, University of Pisa, 2021   %%%%%%%%%%
%%%%%%%%%%%%%%%%%%%%%%%%%%%%%%%%%%%%%%%%%%%%%%%%%%%%%%%%%%%%%%%%%%%%%%%%%%

== matlab function EKF_sim/MATLAB Function ==
  data: or_rad output; u input
% --------------------          quat2ypr            -------------------- %
%{
% This function transform attitude quaternion in Euler angles
%}

function or_rad  = quat2ypr(u)
q = quaternion([u(1) u(2) u(3) u(4)]);
or_rad = [0,0,0]';
or_rad = (euler(q,'zyx','frame'))';
end


%% %%%%%%%%%%%%%%%%%%%%%%%%%%%%%%%%%%%%%%%%%%%%%%%%%%%%%%%%%%%%%%%%%%%%%%%
     %%%%%%%%% Direct EKF for 6D Pose,  Marco Borraccino %%%%%%%%%%
     %%%%%%%%%   SGN Project, University of Pisa, 2021   %%%%%%%%%%
%%%%%%%%%%%%%%%%%%%%%%%%%%%%%%%%%%%%%%%%%%%%%%%%%%%%%%%%%%%%%%%%%%%%%%%%%%

== matlab function EKF_sim/EKF_nb/Initialization task/Initialization task ==
  data: flag_init input; flag_init output; acc input; head input; x0 output; P0 output; buffer input; buffer output; buffer_idx input; buffer_idx output; init_time parameter; acc_variance parameter; Delta2 parameter
% --------------------          EKF_init            -------------------- %
%{
% This function computes the initialization task at the start of the
% simulation. The initial attitude and gyroscope bias is calculated from 
% the mean value of the measurement in period [0,init_time]. 
% The matrix P is also initialized with a estimated attitude 
% covariance, see [27] (R. Munguia and A. Grau, "A Practical Method for 
% Implementing an Attitude and Heading Reference System," International 
% Journal of Advanced Robotic Systems, vol. 11, 2014) for more details.

% Input:
%     flag_init    : flag for initialization task
%     acc          : accelerometer measurement
%     head         : Heading measurement from GPS
%     Delta2       : NED reference system Offset
%     buffer       : buffer for calculate the initial mean valus 
%     buffer_idx   : index of buffer for calculate the initial mean value
%     init_time    : Initial period of time for initialization task 
%     acc_variance : Accelerometer Variance

% Output:
%     flag_init    : flag for initialization task
%     x0           : initial vector state
%     P0           : initial matrix P
%     buffer       : buffer for calculate the initial mean valus 
%     buffer_idx   : index of buffer for calculate the initial mean value
%}
%%
function [flag_init, x0, P0,buffer,buffer_idx] = EKF_init(flag_init, acc,head,buffer,buffer_idx, init_time,acc_variance, Delta2)
    x0 = zeros(16,1);
    P0 = zeros(16,16);
    
    %fill the buffer with initial sensors measurements
    if flag_init == -1
        buffer(buffer_idx,1:3) = -acc;
        buffer(buffer_idx,4) = head;
        buffer_idx = buffer_idx + 1;
    end

    if buffer_idx == 100*init_time && flag_init == -1 %..after [init_time]
        
        %calculate initial value of state variable and matrix P
        g0          = mean(buffer(:,1:3));  
        roll_init   = atan2(g0(2),g0(3));
        pitch_init  = atan2(-g0(1),(g0(2)^2+g0(3)^2)^0.5);
        yaw_init    = pi/2;
%        yaw_init    = mean(buffer(:,4));
        
        q = new_q(yaw_init,pitch_init,roll_init);
        x0 = [  q(1)              q(2)            q(3)            q(4)    ...
                0                 0               0                       ...
                Delta2(2)         Delta2(1)       -Delta2(3)              ...
                0                 0               0                       ...
                0                 0               0                       ]';
        Pq = Pq_init_calculation(roll_init,pitch_init,yaw_init,acc_variance,init_time); 
        P0 = blkdiag(Pq, diag([ 4.8e-6  4.8e-6  4.8e-6          ...
                                1       1       1               ...
                                0.1     0.1     0.1             ...
                                4.8e-2  4.8e-2  4.8e-2          ]));
        flag_init = 1;
    end
end

%% Auxiliary Functions
% This function calculate the initial Pq0, in the same manner as [27].
% % See 'calcolo_matrice_Pq0.m' for the symbolic calculation used.
function Pq = Pq_init_calculation(roll,pitch,yaw,acc_variance,init_time)
    P_ = eye(3)* acc_variance/(init_time*100);
    dq= [                                                                                                                                                                                                                                -(cos(pitch)*sin(roll) + cos(yaw)*sin(roll) - cos(roll)*sin(pitch)*sin(yaw))/(2*(cos(pitch)*cos(roll) + cos(pitch)*cos(yaw) + cos(roll)*cos(yaw) + sin(pitch)*sin(roll)*sin(yaw) + 1)^(1/2)),                                                                                                                                                                                                                        -(cos(roll)*sin(pitch) + cos(yaw)*sin(pitch) - cos(pitch)*sin(roll)*sin(yaw))/(2*(cos(pitch)*cos(roll) + cos(pitch)*cos(yaw) + cos(roll)*cos(yaw) + sin(pitch)*sin(roll)*sin(yaw) + 1)^(1/2)),                                                                                                                                                                                                                                -(cos(pitch)*sin(yaw) + cos(roll)*sin(yaw) - cos(yaw)*sin(pitch)*sin(roll))/(2*(cos(pitch)*cos(roll) + cos(pitch)*cos(yaw) + cos(roll)*cos(yaw) + sin(pitch)*sin(roll)*sin(yaw) + 1)^(1/2));
                   - cos(roll)*cos(yaw) - (cos(pitch)*cos(roll))/(4*(cos(pitch)*cos(roll) + cos(pitch)*cos(yaw) + cos(roll)*cos(yaw) + sin(pitch)*sin(roll)*sin(yaw) + 1)^(1/2)) - sin(pitch)*sin(roll)*sin(yaw) - (cos(pitch)*sin(roll)*(cos(pitch)*sin(roll) + cos(yaw)*sin(roll) - cos(roll)*sin(pitch)*sin(yaw)))/(8*(cos(pitch)*cos(roll) + cos(pitch)*cos(yaw) + cos(roll)*cos(yaw) + sin(pitch)*sin(roll)*sin(yaw) + 1)^(3/2)),                         (sin(pitch)*sin(roll))/(4*(cos(pitch)*cos(roll) + cos(pitch)*cos(yaw) + cos(roll)*cos(yaw) + sin(pitch)*sin(roll)*sin(yaw) + 1)^(1/2)) + cos(pitch)*cos(roll)*sin(yaw) - (cos(pitch)*sin(roll)*(cos(roll)*sin(pitch) + cos(yaw)*sin(pitch) - cos(pitch)*sin(roll)*sin(yaw)))/(8*(cos(pitch)*cos(roll) + cos(pitch)*cos(yaw) + cos(roll)*cos(yaw) + sin(pitch)*sin(roll)*sin(yaw) + 1)^(3/2)),                                                                                                                                                     sin(roll)*sin(yaw) + cos(roll)*cos(yaw)*sin(pitch) - (cos(pitch)*sin(roll)*(cos(pitch)*sin(yaw) + cos(roll)*sin(yaw) - cos(yaw)*sin(pitch)*sin(roll)))/(8*(cos(pitch)*cos(roll) + cos(pitch)*cos(yaw) + cos(roll)*cos(yaw) + sin(pitch)*sin(roll)*sin(yaw) + 1)^(3/2));
          - (cos(roll)*sin(yaw) - cos(yaw)*sin(pitch)*sin(roll))/(4*(cos(pitch)*cos(roll) + cos(pitch)*cos(yaw) + cos(roll)*cos(yaw) + sin(pitch)*sin(roll)*sin(yaw) + 1)^(1/2)) - ((sin(roll)*sin(yaw) + cos(roll)*cos(yaw)*sin(pitch))*(cos(pitch)*sin(roll) + cos(yaw)*sin(roll) - cos(roll)*sin(pitch)*sin(yaw)))/(8*(cos(pitch)*cos(roll) + cos(pitch)*cos(yaw) + cos(roll)*cos(yaw) + sin(pitch)*sin(roll)*sin(yaw) + 1)^(3/2)), - cos(pitch) - ((sin(roll)*sin(yaw) + cos(roll)*cos(yaw)*sin(pitch))*(cos(roll)*sin(pitch) + cos(yaw)*sin(pitch) - cos(pitch)*sin(roll)*sin(yaw)))/(8*(cos(pitch)*cos(roll) + cos(pitch)*cos(yaw) + cos(roll)*cos(yaw) + sin(pitch)*sin(roll)*sin(yaw) + 1)^(3/2)) - (cos(pitch)*cos(roll)*cos(yaw))/(4*(cos(pitch)*cos(roll) + cos(pitch)*cos(yaw) + cos(roll)*cos(yaw) + sin(pitch)*sin(roll)*sin(yaw) + 1)^(1/2)), - (cos(yaw)*sin(roll) - cos(roll)*sin(pitch)*sin(yaw))/(4*(cos(pitch)*cos(roll) + cos(pitch)*cos(yaw) + cos(roll)*cos(yaw) + sin(pitch)*sin(roll)*sin(yaw) + 1)^(1/2)) - ((sin(roll)*sin(yaw) + cos(roll)*cos(yaw)*sin(pitch))*(cos(pitch)*sin(yaw) + cos(roll)*sin(yaw) - cos(yaw)*sin(pitch)*sin(roll)))/(8*(cos(pitch)*cos(roll) + cos(pitch)*cos(yaw) + cos(roll)*cos(yaw) + sin(pitch)*sin(roll)*sin(yaw) + 1)^(3/2));
                                                                                                                                                              sin(roll)*sin(yaw) + cos(roll)*cos(yaw)*sin(pitch) - (cos(pitch)*sin(yaw)*(cos(pitch)*sin(roll) + cos(yaw)*sin(roll) - cos(roll)*sin(pitch)*sin(yaw)))/(8*(cos(pitch)*cos(roll) + cos(pitch)*cos(yaw) + cos(roll)*cos(yaw) + sin(pitch)*sin(roll)*sin(yaw) + 1)^(3/2)),                           (sin(pitch)*sin(yaw))/(4*(cos(pitch)*cos(roll) + cos(pitch)*cos(yaw) + cos(roll)*cos(yaw) + sin(pitch)*sin(roll)*sin(yaw) + 1)^(1/2)) + cos(pitch)*cos(yaw)*sin(roll) - (cos(pitch)*sin(yaw)*(cos(roll)*sin(pitch) + cos(yaw)*sin(pitch) - cos(pitch)*sin(roll)*sin(yaw)))/(8*(cos(pitch)*cos(roll) + cos(pitch)*cos(yaw) + cos(roll)*cos(yaw) + sin(pitch)*sin(roll)*sin(yaw) + 1)^(3/2)),            - cos(roll)*cos(yaw) - (cos(pitch)*cos(yaw))/(4*(cos(pitch)*cos(roll) + cos(pitch)*cos(yaw) + cos(roll)*cos(yaw) + sin(pitch)*sin(roll)*sin(yaw) + 1)^(1/2)) - sin(pitch)*sin(roll)*sin(yaw) - (cos(pitch)*sin(yaw)*(cos(pitch)*sin(yaw) + cos(roll)*sin(yaw) - cos(yaw)*sin(pitch)*sin(roll)))/(8*(cos(pitch)*cos(roll) + cos(pitch)*cos(yaw) + cos(roll)*cos(yaw) + sin(pitch)*sin(roll)*sin(yaw) + 1)^(3/2))];
    Pq = dq*P_*dq';
end

% This function create a quaternion from Euler's angle [Yaw,Pitch,Roll]
function q = new_q(yaw,pitch,roll)
    q = zeros(1,4);
    q(1) = cos(roll/2) * cos(pitch/2) * cos(yaw/2) + sin(roll/2) * sin(pitch/2) * sin(yaw/2);
    q(2) = sin(roll/2) * cos(pitch/2) * cos(yaw/2) - cos(roll/2) * sin(pitch/2) * sin(yaw/2);
    q(3) = cos(roll/2) * sin(pitch/2) * cos(yaw/2) + sin(roll/2) * cos(pitch/2) * sin(yaw/2);
    q(4) = cos(roll/2) * cos(pitch/2) * sin(yaw/2) - sin(roll/2) * sin(pitch/2) * cos(yaw/2);  
end

%% %%%%%%%%%%%%%%%%%%%%%%%%%%%%%%%%%%%%%%%%%%%%%%%%%%%%%%%%%%%%%%%%%%%%%%%
     %%%%%%%%% Direct EKF for 6D Pose,  Marco Borraccino %%%%%%%%%%
     %%%%%%%%%   SGN Project, University of Pisa, 2021   %%%%%%%%%%
%%%%%%%%%%%%%%%%%%%%%%%%%%%%%%%%%%%%%%%%%%%%%%%%%%%%%%%%%%%%%%%%%%%%%%%%%%

== matlab function EKF_sim/MATLAB Function2 ==
  data: pos_ENU input; pos_NED output; Delta2 parameter
% --------------------         ENU2NED_pos           -------------------- %
%{
% This function transform reference position in navigation frame, from ENU
% to NED, passing by the ENU2NED rotation matrix.
%}

function pos_NED = ENU2NED_pos(pos_ENU,Delta2)

    %R_ENU2NED rotation matriX:
    R = [0  1  0; ...
         1  0  0; ...
         0  0 -1];
    pos_NED = (R*[pos_ENU(1)+Delta2(1), pos_ENU(2)+Delta2(2), pos_ENU(3)+Delta2(3)]');
end

%% %%%%%%%%%%%%%%%%%%%%%%%%%%%%%%%%%%%%%%%%%%%%%%%%%%%%%%%%%%%%%%%%%%%%%%%
     %%%%%%%%% Direct EKF for 6D Pose,  Marco Borraccino %%%%%%%%%%
     %%%%%%%%%   SGN Project, University of Pisa, 2021   %%%%%%%%%%
%%%%%%%%%%%%%%%%%%%%%%%%%%%%%%%%%%%%%%%%%%%%%%%%%%%%%%%%%%%%%%%%%%%%%%%%%%%

== matlab function EKF_sim/MATLAB Function6 ==
  data: ypr_ENU input; ypr_NED output
% --------------------         ENU2NED_ypr           -------------------- %
%{
% This function transform attitude angles (yaw,pitch roll) from describing
% rotation from body to NED, instead of body to ENU. This in computed passing
% by the equivalent rotation matrix trasformed by the ENU2NED rotation.
%}

function ypr_NED = ENU2NED_ypr(ypr_ENU)
    ypr_NED = [0;0;0];
    coder.extrinsic('rotm2eul');
    R_body2ENU = calcolo_R(ypr_ENU(1),ypr_ENU(2),ypr_ENU(3));
    R_ENU2NED = [0 1 0; 1 0 0; 0 0 -1];
    R_body2NED = R_ENU2NED*R_body2ENU;
    ypr_NED = rotm2eul(R_body2NED,'zyx');
end

%Body-to-navigation Rotation Matrix from Euler's Angles [Yaw,Pitch,Roll]
function R = calcolo_R(Yaw,Pitch,Roll)
    R_x = [ 1               0              0   ;
            0           cos(Roll)     sin(Roll);
            0           -sin(Roll)    cos(Roll)];
    R_y = [cos(Pitch)       0   -sin(Pitch);
              0             1         0    ;
           sin(Pitch)       0    cos(Pitch)];
    R_z = [cos(Yaw)     sin(Yaw)      0;
          -sin(Yaw)     cos(Yaw)      0;
              0            0          1];
    R = (R_z'*R_y')*R_x';    
end

%% %%%%%%%%%%%%%%%%%%%%%%%%%%%%%%%%%%%%%%%%%%%%%%%%%%%%%%%%%%%%%%%%%%%%%%%
     %%%%%%%%% Direct EKF for 6D Pose,  Marco Borraccino %%%%%%%%%%
     %%%%%%%%%   SGN Project, University of Pisa, 2021   %%%%%%%%%%
%%%%%%%%%%%%%%%%%%%%%%%%%%%%%%%%%%%%%%%%%%%%%%%%%%%%%%%%%%%%%%%%%%%%%%%%%%%

== matlab function EKF_sim/MATLAB Function3 ==
  data: u input; y output
function y = wrap2pi(u)
    y = 0;
    coder.extrinsic('wrapToPi');

    y = wrapToPi(u);
end

== matlab function EKF_sim/EKF_nb/MATLAB Function ==
  data: GPS input; GPS_NED output; lon0 parameter; lat0 parameter; h0 parameter
% --------------------          ECEF2NED            -------------------- %
%{
% This function transform the GPS data from ECEF to NED reference system.
% 'geodetic2ned' function is used with 'wgs84' Earth model.

% Input:
%     GPS         : GPS data [3x1] lat-lon-h [degree,degree,m]
%     lon0        : Origin Longitude of NED
%     lat0        : Origin Latitude of NED
%     h0          : Origin Height of NED

% Output:
%     GPS_NED     : GPS data [3x1] in NED North-East-Down [m]

%}
%%
function GPS_NED = ECEF2NED(GPS,lon0,lat0,h0)
    GPS_NED = [0 0 0];
    coder.extrinsic('evalin', 'wgs84Ellipsoid', 'geodetic2ned');
    [GPS_NED(1),GPS_NED(2),GPS_NED(3)]= geodetic2ned(GPS(1), GPS(2), GPS(3),...
                                                     lat0, lon0, h0, wgs84Ellipsoid,'degree');
end

%% %%%%%%%%%%%%%%%%%%%%%%%%%%%%%%%%%%%%%%%%%%%%%%%%%%%%%%%%%%%%%%%%%%%%%%%
     %%%%%%%%% Direct EKF for 6D Pose,  Marco Borraccino %%%%%%%%%%
     %%%%%%%%%   SGN Project, University of Pisa, 2021   %%%%%%%%%%
%%%%%%%%%%%%%%%%%%%%%%%%%%%%%%%%%%%%%%%%%%%%%%%%%%%%%%%%%%%%%%%%%%%%%%%%%%

== matlab function EKF_sim/EKF_nb/MATLAB Function1 ==
  data: x input; q output; w output; r output; v output; a output
% --------------------         extract_var         -------------------- %
%{
% This function extracts single variables from the state vector.

% Input:
%     x  :  [q w r v a]' state vector [16x1]:

% Output:
%     q  : [q1 q2 q3 q4]     unit quaternion representing the attitude (1 2 3 4)
%     w  : [wx wy wz]        angular velocity (5 6 7)
%     r  : [rx ry rz]        position (NED)(8 9 10)
%     v  : [vx vy vz]        linear velocity (NED) (11 12 13)
%     a  : [ax ay az]        linear acceleration (NED) (14 15 16)
%}
%%
function [q, w, r, v, a] = extract_var(x)
    q  = x(1:4);
    w  = x(5:7);
    r  = x(8:10);
    v  = x(11:13);
    a  = x(14:16);
end

%% %%%%%%%%%%%%%%%%%%%%%%%%%%%%%%%%%%%%%%%%%%%%%%%%%%%%%%%%%%%%%%%%%%%%%%%
     %%%%%%%%% Direct EKF for 6D Pose,  Marco Borraccino %%%%%%%%%%
     %%%%%%%%%   SGN Project, University of Pisa, 2021   %%%%%%%%%%
%%%%%%%%%%%%%%%%%%%%%%%%%%%%%%%%%%%%%%%%%%%%%%%%%%%%%%%%%%%%%%%%%%%%%%%%%%
